simulink model "satellitsimuppgift"  (R2014a)
settings: Solver=ode45  StartTime=0.0  StopTime=55  RelTol=1e-3
libraries: simulink x2
settings Model: Creator=CTGIKO  LastModifiedBy=ad0548
settings DebuggingCC: UnderspecifiedInitializationDetection=Classic

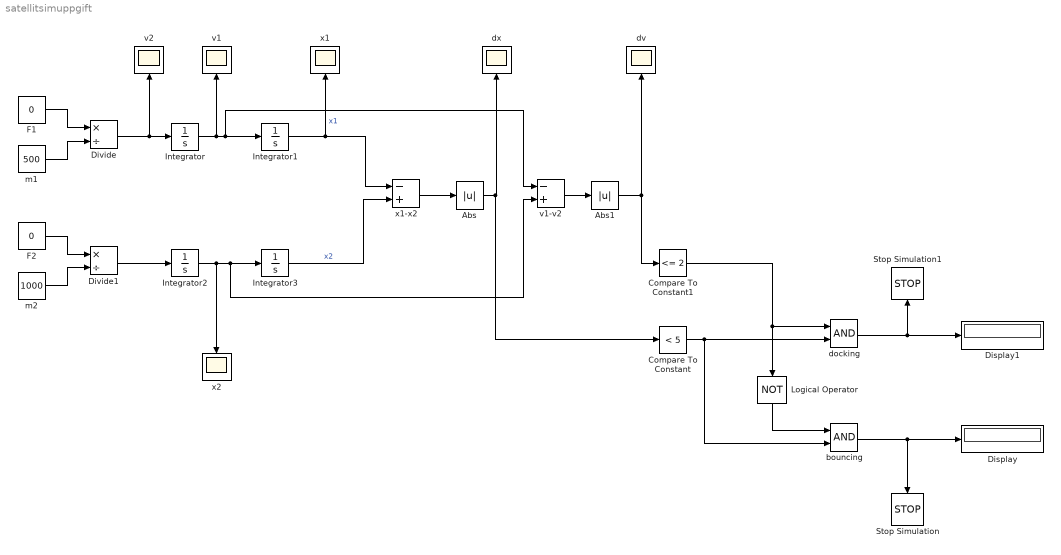
== system satellitsimuppgift ==
  Abs : Abs
  Abs1 : Abs
  Compare To Constant : simulink/Logic and Bit Operations/Compare To Constant  relop=<  const=5  OutDataTypeStr=boolean
  Compare To Constant1 : simulink/Logic and Bit Operations/Compare To Constant  relop=<=  const=2  OutDataTypeStr=boolean
  Display : Display
  Display1 : Display
  Divide : Product  Inputs=*/
  Divide1 : Product  Inputs=*/
  F1 : Constant  Value=0
  F2 : Constant  Value=0
  Integrator : Integrator  InitialCondition=2
  Integrator1 : Integrator
  Integrator2 : Integrator
  Integrator3 : Integrator  InitialCondition=100
  Logical Operator : Logic  Operator=NOT  AllPortsSameDT=off  OutDataTypeStr=boolean
  Stop Simulation : Stop
  Stop Simulation1 : Stop
  bouncing : Logic  AllPortsSameDT=off  OutDataTypeStr=boolean
  docking : Logic  AllPortsSameDT=off  OutDataTypeStr=boolean
  dv : Scope
      settings: YMin=-1000  YMax=100  SaveName=ScopeData4
  dx : Scope
      settings: YMin=5  YMax=50  SaveName=ScopeData2
  m1 : Constant  Value=500
  m2 : Constant  Value=1000
  v1 : Scope
      settings: TimeRange=50  YMin=0  YMax=9  SaveName=ScopeData3
  v1-v2 : Sum  Inputs=-+
  v2 : Scope
      settings: TimeRange=50  YMin=0  YMax=9  SaveName=ScopeData5
  x1 : Scope
  x1-x2 : Sum  Inputs=-+
  x2 : Scope
  wires:
  F1/1 -> Divide/1
  m1/1 -> Divide/2
  F2/1 -> Divide1/1
  m2/1 -> Divide1/2
  Divide/1 -> Integrator/1, v2/1
  Integrator1/1 -> x1-x2/1, x1/1  "x1"
  Divide1/1 -> Integrator2/1
  Integrator2/1 -> x2/1, v1-v2/2, Integrator3/1
  Integrator3/1 -> x1-x2/2  "x2"
  x1-x2/1 -> Abs/1
  v1-v2/1 -> Abs1/1
  Abs/1 -> Compare To Constant/1, dx/1
  Integrator/1 -> v1-v2/1, Integrator1/1, v1/1
  Abs1/1 -> Compare To Constant1/1, dv/1
  Compare To Constant1/1 -> docking/1, Logical Operator/1
  Logical Operator/1 -> bouncing/1
  Compare To Constant/1 -> docking/2, bouncing/2
  bouncing/1 -> Display/1, Stop Simulation/1
  docking/1 -> Display1/1, Stop Simulation1/1
